simulink model "motorcontroller"  (R2015a)
settings: Solver=ode45  StartTime=0.0  StopTime=10.0  RelTol=1e-3
undefined symbols (not defined in the file): Hydride, magnitude, Metal, Nickel, Ts
libraries: powerlib x43, simulink_extras x8, driveline x4, electricdrivelib x3, simulink x2, powerlib_extras x2, DC6DriveInternalModels x1
(part 1 of 2)
settings Model: Creator=Elena  LastModifiedBy=Elena

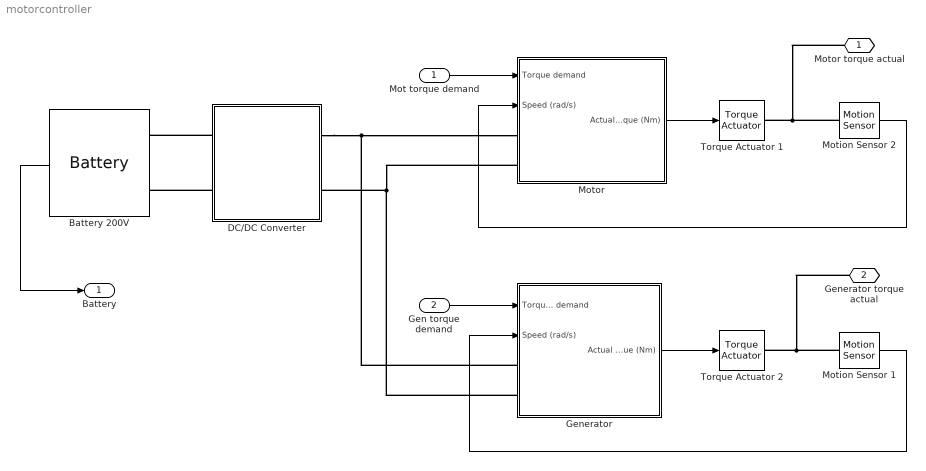
== system motorcontroller ==
  Mot torque demand : Inport
  Gen torque demand : Inport  Port=2
  Battery 200V : electricdrivelib/Extra Sources/Battery  BatType=Nickel-Metal-Hydride  ShowDetailedParameters=off  NomV=200  NomQ=6.5  SOC=final_SOC(end)  PresetModel=on  MaxQ=7  FullV=235.5932  Dis_rate=1.3  R=0.30769  Normal_OP=6.25  expZone="[216.9492           1.3]"  current=[50 100]  Units=Time  Batt_Tr=30
  DC/DC Converter : Subsystem
      mask init:
      | [X1,X1m,X2,X2m,X3,X4,Y1,Y1m,Y2,Y2m,Y3,Y4,color1,color2]=spsdrivelogo;
      mask Display:
      | patch([X1 X1m],[Y1 Y1m],color1);
      | patch(X3,Y3,color2);
      | plot([X1 X1m X2 X2m X3 X4],[Y1 Y1m Y2 Y2m Y3 Y4]);
  "Generator " : Subsystem
  Motion Sensor 1 : driveline/Sensors & Actuators/Motion Sensor  Angle=off  x0=0  Velocity=on  Acceleration=off
  Motion Sensor 2 : driveline/Sensors & Actuators/Motion Sensor  Angle=off  x0=0  Velocity=on  Acceleration=off
  Motor : Subsystem
  Torque Actuator 1 : driveline/Sensors & Actuators/Torque Actuator
  Torque Actuator 2 : driveline/Sensors & Actuators/Torque Actuator
  Motor torque actual : PMIOPort  Port=1  Side=Left
  Generator torque actual : PMIOPort  Port=2  Side=Right
  Battery : Outport
  wires:
  Battery 200V/1 -> Battery/1
  Mot torque demand/1 -> Motor/1(Torque demand)
  Gen torque demand/1 -> "Generator "/1(Torque demand)
  Motion Sensor 1/1 -> "Generator "/2(Speed (rad/s))
  Motor/1(Actual torque (Nm)) -> Torque Actuator 1/1
  "Generator "/1(Actual torque (Nm)) -> Torque Actuator 2/1
  Motion Sensor 2/1 -> Motor/2(Speed (rad/s))
  connections:
  DC/DC Converter/LConn1 -- Battery 200V/LConn1
  DC/DC Converter/LConn2 -- Battery 200V/LConn2
  DC/DC Converter/RConn1 -- "Generator "/LConn1 -- Motor/LConn1
  Motor/LConn2 -- "Generator "/LConn2 -- DC/DC Converter/RConn2
  Motor torque actual/RConn1 -- Motion Sensor 2/LConn1 -- Torque Actuator 1/RConn1
  Generator torque actual/RConn1 -- Torque Actuator 2/RConn1 -- Motion Sensor 1/LConn1

== system motorcontroller/DC//DC Converter ==
  Bus DC controller : Subsystem
  DC/DC converter : Subsystem
  Ubus Ref : Constant  Value=500
  +Vdc Bus : PMIOPort  Tag=PMCPort  Port=1  Side=Right
  -Vdc Bus : PMIOPort  Tag=PMCPort  Port=2  Side=Right
  + battery : PMIOPort  Tag=PMCPort  Port=3  Side=Left
  - battery : PMIOPort  Tag=PMCPort  Port=4  Side=Left
  wires:
  Ubus Ref/1 -> Bus DC controller/2(Uref)
  Bus DC controller/1(Duty cycle) -> DC/DC converter/1(Duty Cycle)
  DC/DC converter/1(UBus) -> Bus DC controller/1(Ubus)
  connections:
  +Vdc Bus/RConn1 -- DC/DC converter/LConn1
  -Vdc Bus/RConn1 -- DC/DC converter/LConn2
  + battery/RConn1 -- DC/DC converter/RConn1
  - battery/RConn1 -- DC/DC converter/RConn2

== system motorcontroller/Generator  ==
  Torque demand : Inport
  Speed (rad/s) : Inport  Port=2
  Bus Selector : BusSelector  OutputSignals=Rotor speed wm (rad/s),Rotor angle thetam (rad),Electromagnetic torque Te (N*m)
  Measures : electricdrivelib/AC drives/PM Synchronous Motor Drive/Measures
  Mux : Subsystem
  PMSM1 : powerlib/Machines/Permanent Magnet Synchronous Machine  NbPhases=3  FluxDistribution=Sinusoidal  RotorType=Salient-pole  MechanicalLoad=Speed w  PresetModel=No  ShowDetailedParameters=on  MeasurementBus=off  Resistance=0.05  Inductance=0  dqInductances=[0.000635 0.000635]  La=0.000835  MachineConstant=Flux linkage established by magnets (V.s)  Flux=0.192  VoltageCst=34.8249  TorqueCst=0.288  Flat=0  Mechanical=[0.011 0.001889/4 4/4]  PolePairs=1  InitialConditions=[0,0, 0,0,0]  InitialConditions5ph=[0 0 0 0 0 0]  TsPowergui=0  TsBlock=-1  RefAngle=90 degrees behind phase A axis (modified Park)
      settings: AttributesFormatString=\n
  Speed Controller : Subsystem  mask(Speed controller){SwK=Torque regulation, bs=1800, ramp=[-5000,5000], kp=(1/5)/4, ki=(50/5)/4/3, fc=(1000/10)/2, ctrl_sat=[-45,45], Tsc=Ts}
      mask prompts: SwK "Regulation type"; bs "Base speed (rpm)"; ramp "Speed reference ramp (rpm/s) [deceleration,acceleration]"; kp "Proportional gain"; ki "Integral gain"; fc "Speed measurement - low-pass filter cutoff frequency (Hz)"; ctrl_sat "Controller output torque saturation (N.m) [negative,positive]"; Tsc "Controller sampling time (s)"
      mask help: This block implements a PI speed regulator.
      mask init:
      | [X1,X1m,X2,X2m,X3,X4,Y1,Y1m,Y2,Y2m,Y3,Y4,color1,color2]=spsdrivelogo;
      mask TypeOptions SwK: Speed regulation | Torque regulation
      mask Display:
      | patch([X1 X1m],[Y1 Y1m],color1);
      | patch(X3,Y3,color2);
      | plot([X1 X1m X2 X2m X3 X4],[Y1 Y1m Y2 Y2m Y3 Y4]);
  Three-phase Inverter : Subsystem  mask(SPSdrives Converter){Arms=3, SnubberResistance=5000, SnubberCapacitance=inf, Device=IGBT / Diodes, Ron=1e-3, Lon=0, ForwardVoltages=[0.8,0.8], ForwardVoltage=0, GTOparameters=[0,0], IGBTparameters=[1e-6,2e-6], Measurements=All voltages and currents, SourceFrequency=60, dqInductances=[0.000635,0.000635], Flux=0.192, Resistance=0.05, p=4/4, converterType=Inverter}
      mask prompts: Arms "Number of bridge arms:"; SnubberResistance "Snubber resistance Rs (Ohms)"; SnubberCapacitance "Snubber capacitance Cs (F)"; Device "Power Electronic device"; Ron "Ron (Ohms)"; Lon "Lon (H)"; ForwardVoltages "Forward voltages  [ Device Vf(V) , Diode Vfd(V)]"; ForwardVoltage "Forward voltage Vf (V)"; GTOparameters "[  Tf (s) , Tt (s)  ]"; IGBTparameters "[  Tf (s) , Tt (s)  ]"; SourceFrequency "Source Frequency (Hz)"; dqInductances "PMSM-Inductances [ Ld(H) Lq(H) ]:"; Flux "PMSM-Flux induced by magnets (Wb):"; Resistance "PMSM-Stator resistance Rs (ohm):"; p "PMSM-Pairs of poles p:"; converterType "Converter type:"
      mask init:
      | Ld=dqInductances(1);
      | Lq=dqInductances(2);
      | Fcs=6*SourceFrequency/10;
      settings: OpenFcn=power_openblockproxy();
      mask Help: web(psbhelp);
      mask TypeOptions Arms: 1 | 2 | 3
      mask TypeOptions Device: Diodes | Thyristors | GTO / Diodes | MOSFET / Diodes | IGBT / Diodes | Ideal Switches
      mask TypeOptions Measurements: None | Device voltages | Device currents | UAB UBC UCA UDC voltages | All voltages and currents
      mask TypeOptions converterType: Rectifier | Inverter
      mask Display: plot(0,0,100,100,[39 39 23.8],[71 28 28],[44 56 49.6 56 52.8 56 61 61],[39.2 33.6 32.8 33.6 40.8 33.6 30 12.4],[44 44 44 61 61],[28 71 60 66.4 90],[75 67 83 75 67 83 75 75],[54 42 42 54 54 54 54 66],[61 75 75],[24 24 42],[75 75 61],[66,76,76])
  VECT : Subsystem  mask(VECT){nb_p=4/4, lambda=0.192, freq_max=20e3, Ts_vect=Ts, h=2}
      mask prompts: nb_p "Motor pairs of poles"; lambda "Flux induced by magnets (Wb)"; freq_max "Maximum switching frequency (Hz)"; Ts_vect "Sampling time (s)"; h "Current hysteresis bandwidth (A)"
      mask help: This block implements a vector controller.
      mask init:
      | [X1,X1m,X2,X2m,X3,X4,Y1,Y1m,Y2,Y2m,Y3,Y4,color1,color2]=spsdrivelogo;
      mask Display:
      | patch([X1 X1m],[Y1 Y1m],color1);
      | patch(X3,Y3,color2);
      | plot([X1 X1m X2 X2m X3 X4],[Y1 Y1m Y2 Y2m Y3 Y4]);
  + : PMIOPort  Port=1  Side=Left
  - : PMIOPort  Port=2  Side=Left
  Actual torque (Nm) : Outport
  wires:
  ? -> VECT/1(En), Speed Controller/3(En)
  Torque demand/1 -> Speed Controller/2(N*)
  Speed Controller/1(Torque*) -> VECT/2(Torque*)
  Bus Selector/1 -> Speed Controller/1(N)  "<Rotor speed wm (rad/s)>"
  PMSM1/1 -> Mux/2(m), Bus Selector/1
  Speed (rad/s)/1 -> PMSM1/1
  Bus Selector/3 -> Actual torque (Nm)/1  "<Electromagnetic torque Te (N*m)>"
  Measures/1 -> VECT/4(I_abc)
  Speed Controller/2(Ctrl) -> ?
  VECT/1(sig*) -> Mux/1(sig*)
  Mux/1(Ctrl) -> Three-phase Inverter/1(ctrl)
  Bus Selector/2 -> VECT/3(teta)  "<Rotor angle thetam (rad)>"
  connections:
  -/RConn1 -- Three-phase Inverter/RConn2
  +/RConn1 -- Three-phase Inverter/RConn1
  Measures/RConn1 -- PMSM1/LConn1
  Measures/RConn2 -- PMSM1/LConn2
  Measures/RConn3 -- PMSM1/LConn3
  Three-phase Inverter/LConn1 -- Measures/LConn1
  Measures/LConn2 -- Three-phase Inverter/LConn2
  Three-phase Inverter/LConn3 -- Measures/LConn3

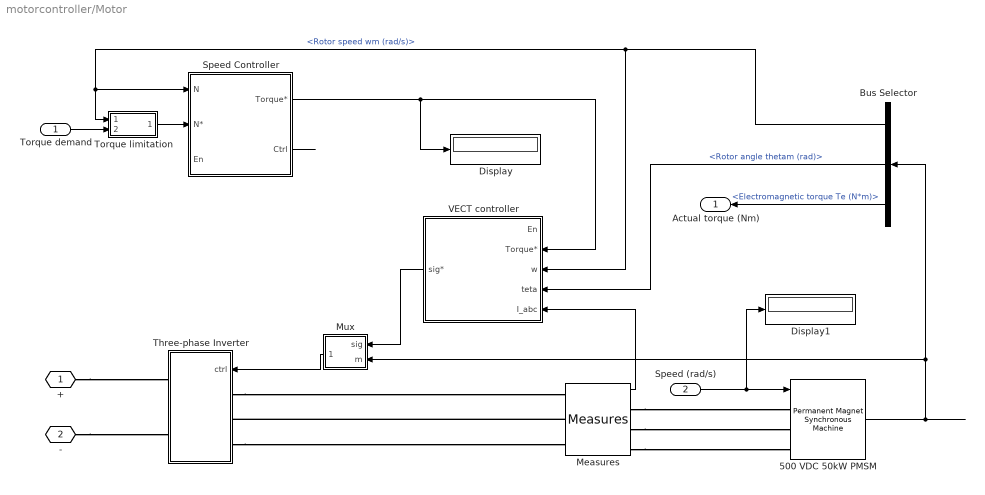
== system motorcontroller/Motor ==
  Torque demand : Inport
  Speed (rad/s) : Inport  Port=2
  500 VDC 50kW PMSM : powerlib/Machines/Permanent Magnet Synchronous Machine  NbPhases=3  FluxDistribution=Sinusoidal  RotorType=Salient-pole  MechanicalLoad=Speed w  PresetModel=No  ShowDetailedParameters=on  MeasurementBus=off  Resistance=0.0065  Inductance=0  dqInductances="[0.001597972349731   0.002057052250467]"  La=0.000835  MachineConstant=Flux linkage established by magnets (V.s)  Flux=0.175666143629361  VoltageCst=127.4493  TorqueCst=1.054  Flat=0  Mechanical=[0.089 0.005 4]  PolePairs=4  InitialConditions=[0,0,0,0]  InitialConditions5ph=[0 0 0 0 0 0]  TsPowergui=0  TsBlock=-1  RefAngle=90 degrees behind phase A axis (modified Park)
      settings: AttributesFormatString=\n
  Bus Selector : BusSelector  OutputSignals=Rotor speed wm (rad/s),Rotor angle thetam (rad),Electromagnetic torque Te (N*m)
  Display : Display
      settings: Decimation=100
  Display1 : Display
      settings: Decimation=100
  Measures : electricdrivelib/AC drives/PM Synchronous Motor Drive/Measures
  Mux : Subsystem
  Speed Controller : Subsystem  mask(Speed controller){SwK=Torque regulation, bs=3000, ramp=[-10000,10000], kp=1/5, ki=50/5, fc=1000/10, ctrl_sat=[-400,400], Tsc=120e-6}
      mask prompts: SwK "Regulation type"; bs "Base speed (rpm)"; ramp "Speed reference ramp (rpm/s) [deceleration,acceleration]"; kp "Proportional gain"; ki "Integral gain"; fc "Speed measurement - low-pass filter cutoff frequency (Hz)"; ctrl_sat "Controller output torque saturation (N.m) [negative,positive]"; Tsc "Controller sampling time (s)"
      mask help: This block implements a PI speed regulator.
      mask init:
      | [X1,X1m,X2,X2m,X3,X4,Y1,Y1m,Y2,Y2m,Y3,Y4,color1,color2]=spsdrivelogo;
      mask TypeOptions SwK: Speed regulation | Torque regulation
      mask Display:
      | patch([X1 X1m],[Y1 Y1m],color1);
      | patch(X3,Y3,color2);
      | plot([X1 X1m X2 X2m X3 X4],[Y1 Y1m Y2 Y2m Y3 Y4]);
  Three-phase Inverter : Subsystem  mask(SPSdrives Converter){Arms=3, SnubberResistance=5000, SnubberCapacitance=inf, Device=IGBT / Diodes, Ron=1e-3, Lon=0, ForwardVoltages=[0.8,0.8], ForwardVoltage=0, GTOparameters=[0,0], IGBTparameters=[1e-6,2e-6], Measurements=All voltages and currents, SourceFrequency=60, dqInductances=[0.001597972349731   0.002057052250467], Flux=0.175666143629361, Resistance=0.0065, p=4, converterType=Inverter}
      mask prompts: Arms "Number of bridge arms:"; SnubberResistance "Snubber resistance Rs (Ohms)"; SnubberCapacitance "Snubber capacitance Cs (F)"; Device "Power Electronic device"; Ron "Ron (Ohms)"; Lon "Lon (H)"; ForwardVoltages "Forward voltages  [ Device Vf(V) , Diode Vfd(V)]"; ForwardVoltage "Forward voltage Vf (V)"; GTOparameters "[  Tf (s) , Tt (s)  ]"; IGBTparameters "[  Tf (s) , Tt (s)  ]"; SourceFrequency "Source Frequency (Hz)"; dqInductances "PMSM-Inductances [ Ld(H) Lq(H) ]:"; Flux "PMSM-Flux induced by magnets (Wb):"; Resistance "PMSM-Stator resistance Rs (ohm):"; p "PMSM-Pairs of poles p:"; converterType "Converter type:"
      mask init:
      | Ld=dqInductances(1);
      | Lq=dqInductances(2);
      | Fcs=6*SourceFrequency/10;
      settings: OpenFcn=power_openblockproxy();
      mask Help: web(psbhelp);
      mask TypeOptions Arms: 1 | 2 | 3
      mask TypeOptions Device: Diodes | Thyristors | GTO / Diodes | MOSFET / Diodes | IGBT / Diodes | Ideal Switches
      mask TypeOptions Measurements: None | Device voltages | Device currents | UAB UBC UCA UDC voltages | All voltages and currents
      mask TypeOptions converterType: Rectifier | Inverter
      mask Display: plot(0,0,100,100,[39 39 23.8],[71 28 28],[44 56 49.6 56 52.8 56 61 61],[39.2 33.6 32.8 33.6 40.8 33.6 30 12.4],[44 44 44 61 61],[28 71 60 66.4 90],[75 67 83 75 67 83 75 75],[54 42 42 54 54 54 54 66],[61 75 75],[24 24 42],[75 75 61],[66,76,76])
  Torque limitation : Subsystem
      mask Display: plot([0;1800;2000;2500;3000;3500], [1;1;0.90*1;0.72*1;0.6*1;0.51*1])
  VECT controller : Subsystem  mask(VECT){nb_p=4, dqInductances=[0.001597972349731   0.002057052250467], lambda=0.175666143629361, Ts_vect=60e-6}
      mask prompts: nb_p "Motor pairs of poles"; dqInductances "Inductances [ Ld(H) Lq(H) ]:"; lambda "Flux induced by magnets (Wb)"; Ts_vect "Sampling time (s)"
      mask help: This block implements a vector controller.
      mask init:
      | [X1,X1m,X2,X2m,X3,X4,Y1,Y1m,Y2,Y2m,Y3,Y4,color1,color2]=spsdrivelogo;
      | ib = lambda/(dqInductances(2)-dqInductances(1));
      | Teb = 3/2*nb_p*lambda*ib;
      | Ld = dqInductances(1);
      | Lq = dqInductances(2);
      | lam = lambda;
      | p=nb_p;
      | ib = lam/(Lq-Ld);
      | iqn = 0:0.01:3;
      | ten = iqn/2.*(sqrt(4*iqn.*iqn+1)+1);
      mask Display:
      | patch([X1 X1m],[Y1 Y1m],color1);
      | patch(X3,Y3,color2);
      | plot([X1 X1m X2 X2m X3 X4],[Y1 Y1m Y2 Y2m Y3 Y4]);
  + : PMIOPort  Port=1  Side=Left
  - : PMIOPort  Port=2  Side=Left
  Actual torque (Nm) : Outport
  wires:
  Mux/1(Ctrl) -> Three-phase Inverter/1(ctrl)
  VECT controller/1(sig*) -> Mux/1(sig)
  Speed Controller/2(Ctrl) -> ?
  Speed (rad/s)/1 -> Display1/1, 500 VDC 50kW PMSM/1
  500 VDC 50kW PMSM/1 -> Bus Selector/1, Mux/2(m)
  Bus Selector/3 -> Actual torque (Nm)/1  "<Electromagnetic torque Te (N*m)>"
  Bus Selector/1 -> VECT controller/3(w), Speed Controller/1(N), Torque limitation/1(N rad/s)  "<Rotor speed wm (rad/s)>"
  ? -> VECT controller/1(En), Speed Controller/3(En)
  Speed Controller/1(Torque*) -> Display/1, VECT controller/2(Torque*)
  Measures/1 -> VECT controller/5(I_abc)
  Bus Selector/2 -> VECT controller/4(teta)  "<Rotor angle thetam (rad)>"
  Torque limitation/1(torque) -> Speed Controller/2(N*)
  Torque demand/1 -> Torque limitation/2(Torque)
  connections:
  Three-phase Inverter/LConn3 -- Measures/LConn3
  Measures/LConn2 -- Three-phase Inverter/LConn2
  Three-phase Inverter/LConn1 -- Measures/LConn1
  Measures/RConn3 -- 500 VDC 50kW PMSM/LConn3
  Measures/RConn2 -- 500 VDC 50kW PMSM/LConn2
  Measures/RConn1 -- 500 VDC 50kW PMSM/LConn1
  +/RConn1 -- Three-phase Inverter/RConn1
  -/RConn1 -- Three-phase Inverter/RConn2

== system motorcontroller/DC//DC Converter/Bus DC controller ==
  Ubus : Inport
  Uref : Inport  Port=2
  Current controller DISCRETE1 : Subsystem  mask(PI controller){Kp=0.001, Ki=1, Ts=Ts}
      mask prompts: Kp "Proportional gain (Kp)"; Ki "Integral gain (Ki)"; Ts "Sample time (s) :"
      mask help: Proportional-Integral Speed Controller
      mask Display: plot(0,0,100,100,[35,35,65],[70,30,30],[35,65],[45,60])
  Display : Display
      settings: Decimation=100
  Duty Cycles : Subsystem
  Mux : Mux  Inputs=2
  Unit Delay2 : UnitDelay  InitialCondition=.5  SampleTime=Ts
  Zero-Order Hold1 : ZeroOrderHold  SampleTime=Ts
  Duty cycle : Outport  InitialOutput=0
  tag scope: V_DCDC=global
  wires:
  Ubus/1 -> Mux/2, Zero-Order Hold1/1
  Mux/1 -> [V_DCDC]
  Uref/1 -> Current controller DISCRETE1/2(Uref), Mux/1
  Current controller DISCRETE1/1(Ec) -> Duty Cycles/1(Ec)
  Zero-Order Hold1/1 -> Display/1, Current controller DISCRETE1/1(UBus)
  Duty Cycles/1(dc) -> Unit Delay2/1
  Unit Delay2/1 -> Duty cycle/1

== system motorcontroller/DC//DC Converter/DC//DC converter ==
  Duty Cycle : Inport
  CBus : powerlib/Elements/Series RLC Branch  LConnTagsString=__new0  RConnTagsString=__new0  BranchType=RC  Resistance=0.2  Inductance=1e-3  SetiL0=off  InitialCurrent=0  Capacitance=1130e-6  Setx0=on  InitialVoltage=500  Measurements=None
  CBus1 : powerlib/Elements/Series RLC Branch  LConnTagsString=__new0  RConnTagsString=__new0  BranchType=C  Resistance=0.2  Inductance=1e-3  SetiL0=off  InitialCurrent=0  Capacitance=282e-6  Setx0=on  InitialVoltage=150  Measurements=None
  Chopper : DC6DriveInternalModels/Chopper (average model)  SnubberResistance=10e3  SnubberCapacitance=inf  Ron=1e-3  ForwardVoltages=[1.3,1.3]  IGBTParameters=[0,0]  converterType=Inverter
  L : powerlib/Elements/Series RLC Branch  LConnTagsString=__new0  RConnTagsString=__new0  BranchType=L  Resistance=0.3  Inductance=373e-6  SetiL0=off  InitialCurrent=100  Capacitance=100e-6  Setx0=off  InitialVoltage=0  Measurements=None
  Neutral2 : powerlib/Elements/Neutral  LConnTagsString=a  NodeNumber=10
  V1 : powerlib/Measurements/Voltage Measurement  PhasorSimulation=off  OutputType=Complex  PSBequivalent=0
  + : PMIOPort  Tag=PMCPort  Port=1  Side=Left
  - : PMIOPort  Tag=PMCPort  Port=2  Side=Left
  + bat. : PMIOPort  Tag=PMCPort  Port=3  Side=Right
  - bat. : PMIOPort  Tag=PMCPort  Port=4  Side=Right
  UBus : Outport
  wires:
  Duty Cycle/1 -> Chopper/1
  V1/1 -> UBus/1
  connections:
  Chopper/RConn1 -- L/RConn1
  L/LConn1 -- + bat./RConn1 -- CBus1/LConn1
  CBus1/RConn1 -- - bat./RConn1 -- Chopper/LConn2 -- -/RConn1 -- CBus/RConn1 -- V1/LConn2 -- Neutral2/LConn1
  +/RConn1 -- CBus/LConn1 -- Chopper/LConn1 -- V1/LConn1

== system motorcontroller/Generator /Mux ==
  sig* : Inport
  m : Inport  Port=2
  Bus Creator : BusCreator  Inputs=2
  Ctrl : Outport
  wires:
  m/1 -> Bus Creator/2  "m"
  sig*/1 -> Bus Creator/1  "Signals*"
  Bus Creator/1 -> Ctrl/1

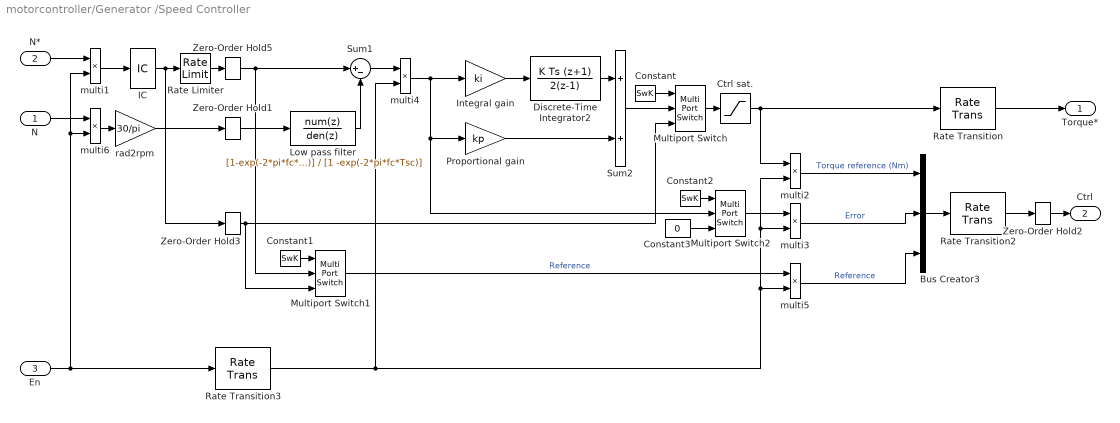
== system motorcontroller/Generator /Speed Controller ==
  N : Inport
  N* : Inport  Port=2
  En : Inport  Port=3
  Bus Creator3 : BusCreator  Inputs=3
  Constant : Constant  Value=SwK
  Constant1 : Constant  Value=SwK
  Constant2 : Constant  Value=SwK
  Constant3 : Constant  Value=0
  Ctrl sat. : Saturate  UpperLimit=ctrl_sat(2)  LowerLimit=ctrl_sat(1)
  Discrete-Time Integrator2 : DiscreteIntegrator  IntegratorMethod=Integration: Trapezoidal  SampleTime=Tsc  LimitOutput=on  UpperSaturationLimit=ctrl_sat(2)  LowerSaturationLimit=ctrl_sat(1)
  IC : InitialCondition  Value=0
  Integral gain : Gain  Gain=ki  SaturateOnIntegerOverflow=on  OutDataTypeStr=Inherit: Same as input  ParamDataTypeStr=Inherit: Same as input
  Low pass filter : DiscreteTransferFcn  Numerator=[1-exp(-2*pi*fc*Tsc)]  Denominator=[1 -exp(-2*pi*fc*Tsc)]  SampleTime=Tsc
  Multiport Switch : MultiPortSwitch  Inputs=2  SaturateOnIntegerOverflow=on
  Multiport Switch1 : MultiPortSwitch  Inputs=2  SaturateOnIntegerOverflow=on
  Multiport Switch2 : MultiPortSwitch  Inputs=2  SaturateOnIntegerOverflow=on
  Proportional gain : Gain  Gain=kp  SaturateOnIntegerOverflow=on  OutDataTypeStr=Inherit: Same as input  ParamDataTypeStr=Inherit: Same as input
  Rate Limiter : RateLimiter  RisingSlewLimit=ramp(2)  FallingSlewLimit=ramp(1)  LinearizeAsGain=off
  Rate Transition : RateTransition
  Rate Transition2 : RateTransition
  Rate Transition3 : RateTransition
  Sum1 : Sum  Inputs=|+-  SaturateOnIntegerOverflow=on  InputSameDT=on  OutDataTypeStr=Inherit: Same as first input
  Sum2 : Sum  SaturateOnIntegerOverflow=on  InputSameDT=on  OutDataTypeStr=Inherit: Same as first input
  Zero-Order Hold1 : ZeroOrderHold  SampleTime=Tsc
  Zero-Order Hold2 : ZeroOrderHold  SampleTime=Ts
  Zero-Order Hold3 : ZeroOrderHold  SampleTime=Tsc
  Zero-Order Hold5 : ZeroOrderHold  SampleTime=Tsc
  multi{1..6} (6 alike) : Product
  rad2rpm : Gain  Gain=30/pi  SaturateOnIntegerOverflow=on  OutDataTypeStr=Inherit: Same as input  ParamDataTypeStr=Inherit: Same as input
  Torque* : Outport
  Ctrl : Outport  Port=2
  wires:
  N/1 -> multi6/1
  multi6/1 -> rad2rpm/1
  N*/1 -> multi1/1
  multi1/1 -> IC/1
  Rate Transition3/1 -> multi5/2, multi2/2, multi3/2, multi4/2
  multi4/1 -> Multiport Switch2/2, Proportional gain/1, Integral gain/1
  Low pass filter/1 -> Sum1/2
  multi2/1 -> Bus Creator3/1  "Torque reference (Nm)"
  Multiport Switch1/1 -> multi5/1  "Reference"
  multi5/1 -> Bus Creator3/3  "Reference"
  multi3/1 -> Bus Creator3/2  "Error"
  Multiport Switch2/1 -> multi3/1
  Zero-Order Hold2/1 -> Ctrl/1
  Rate Transition/1 -> Torque*/1
  En/1 -> multi6/2, multi1/2, Rate Transition3/1
  rad2rpm/1 -> Zero-Order Hold1/1
  Constant3/1 -> Multiport Switch2/3
  Constant2/1 -> Multiport Switch2/1
  Zero-Order Hold3/1 -> Multiport Switch1/3, Multiport Switch/3
  Constant1/1 -> Multiport Switch1/1
  Sum2/1 -> Multiport Switch/2
  Constant/1 -> Multiport Switch/1
  Multiport Switch/1 -> Ctrl sat./1
  Zero-Order Hold5/1 -> Multiport Switch1/2, Sum1/1
  Rate Limiter/1 -> Zero-Order Hold5/1
  Bus Creator3/1 -> Rate Transition2/1
  Rate Transition2/1 -> Zero-Order Hold2/1
  Zero-Order Hold1/1 -> Low pass filter/1
  IC/1 -> Zero-Order Hold3/1, Rate Limiter/1
  Proportional gain/1 -> Sum2/2
  Discrete-Time Integrator2/1 -> Sum2/1
  Sum1/1 -> multi4/1
  Integral gain/1 -> Discrete-Time Integrator2/1
  Ctrl sat./1 -> multi2/1, Rate Transition/1

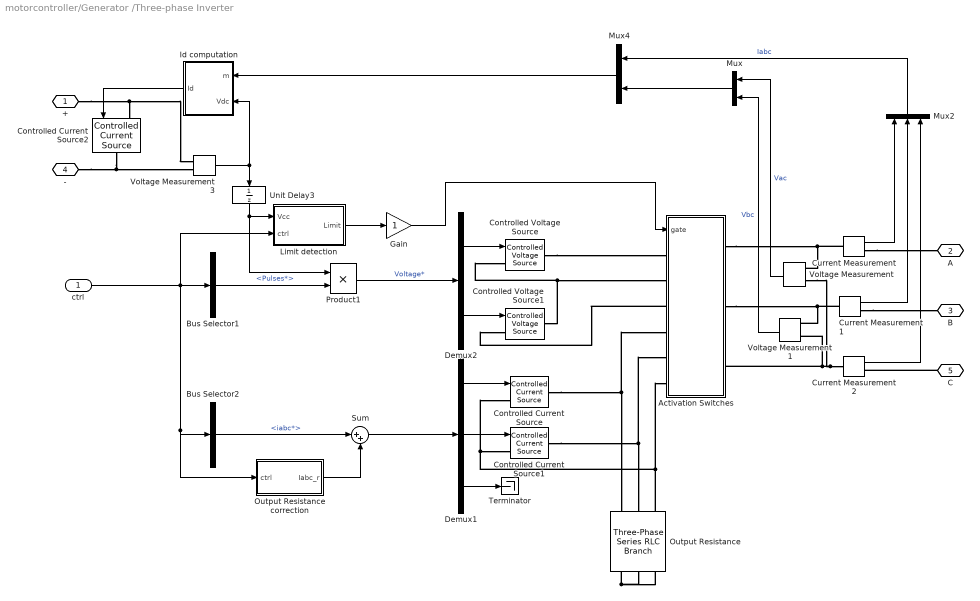
== system motorcontroller/Generator /Three-phase Inverter ==
  ctrl : Inport
  Activation Switches : Subsystem
  Bus Selector1 : BusSelector  OutputSignals=Signals*.Pulses*
  Bus Selector2 : BusSelector  OutputSignals=Signals*.iabc*
  Controlled Current Source : powerlib/Electrical Sources/Controlled Current Source  Initialize=on  Source_Type=AC  Amplitude=0  Phase=0  Frequency=0  Measurements=None
  Controlled Current Source1 : powerlib/Electrical Sources/Controlled Current Source  Initialize=on  Source_Type=AC  Amplitude=0  Phase=0  Frequency=0  Measurements=None
  Controlled Current Source2 : powerlib/Electrical Sources/Controlled Current Source  Initialize=on  Source_Type=AC  Amplitude=0  Phase=0  Frequency=0  Measurements=None
  Controlled Voltage Source : powerlib/Electrical Sources/Controlled Voltage Source  Initialize=on  Source_Type=AC  Amplitude=0  Phase=0  Frequency=0  Measurements=None
  Controlled Voltage Source1 : powerlib/Electrical Sources/Controlled Voltage Source  Initialize=on  Source_Type=AC  Amplitude=0  Phase=0  Frequency=0  Measurements=None
  Current Measurement : powerlib/Measurements/Current Measurement  PhasorSimulation=off  OutputType=Complex  PSBequivalent=0
  Current Measurement1 : powerlib/Measurements/Current Measurement  PhasorSimulation=off  OutputType=Complex  PSBequivalent=0
  Current Measurement2 : powerlib/Measurements/Current Measurement  PhasorSimulation=off  OutputType=Complex  PSBequivalent=0
  Demux1 : Demux  Outputs=3
  Demux2 : Demux  Outputs=2
  Gain : Gain
  Id computation : Subsystem
  Limit detection : Subsystem
  Mux : Mux  Inputs=2
  Mux2 : Mux  Inputs=3
  Mux4 : Mux  Inputs=2
  Output Resistance : powerlib/Elements/Three-Phase Series RLC Branch  LConnTagsString=A|B|C  RConnTagsString=A|B|C  BranchType=R  Resistance=100*Resistance  Inductance=1e-3  Capacitance=1e-6  Measurements=Branch voltages and currents
  Output Resistance correction : Subsystem
  Product1 : Product  RndMeth=Zero
  Sum : Sum  Inputs=|++
  Terminator : Terminator
  Unit Delay3 : UnitDelay  SampleTime=Ts
  Voltage Measurement : powerlib/Measurements/Voltage Measurement  PhasorSimulation=off  OutputType=Complex  PSBequivalent=0
  Voltage Measurement1 : powerlib/Measurements/Voltage Measurement  PhasorSimulation=off  OutputType=Complex  PSBequivalent=0
  Voltage Measurement3 : powerlib/Measurements/Voltage Measurement  PhasorSimulation=off  OutputType=Complex  PSBequivalent=0
  + : PMIOPort  Port=1  Side=Right
  A : PMIOPort  Port=2  Side=Left
  B : PMIOPort  Port=3  Side=Left
  - : PMIOPort  Port=4  Side=Right
  C : PMIOPort  Port=5  Side=Left
  wires:
  Gain/1 -> Activation Switches/1(gate)
  Output Resistance correction/1("Iabc_r ") -> Sum/2
  Product1/1 -> Demux2/1  "Voltage*"
  ctrl/1 -> Output Resistance correction/1(ctrl), Bus Selector2/1, Limit detection/2(ctrl), Bus Selector1/1
  Unit Delay3/1 -> Limit detection/1(Vcc), Product1/1
  Sum/1 -> Demux1/1
  Limit detection/1(Limit) -> Gain/1
  Bus Selector2/1 -> Sum/1  "<iabc*>"
  Demux2/1 -> Controlled Voltage Source/1
  Demux2/2 -> Controlled Voltage Source1/1
  Demux1/3 -> Terminator/1
  Demux1/2 -> Controlled Current Source1/1
  Demux1/1 -> Controlled Current Source/1
  Bus Selector1/1 -> Product1/2  "<Pulses*>"
  Voltage Measurement3/1 -> Id computation/2(Vdc), Unit Delay3/1
  Id computation/1(Id) -> Controlled Current Source2/1
  Mux2/1 -> Mux4/1  "Iabc"
  Mux4/1 -> Id computation/1(m)
  Current Measurement2/1 -> Mux2/3
  Mux/1 -> Mux4/2
  Voltage Measurement1/1 -> Mux/2  "Vbc"
  Voltage Measurement/1 -> Mux/1  "Vac"
  Current Measurement1/1 -> Mux2/2
  Current Measurement/1 -> Mux2/1
  connections:
  Activation Switches/LConn3 -- Controlled Voltage Source1/LConn1
  Controlled Voltage Source/RConn1 -- Activation Switches/LConn1
  C/RConn1 -- Current Measurement2/RConn1
  Current Measurement1/RConn1 -- B/RConn1
  Current Measurement/RConn1 -- A/RConn1
  Current Measurement1/LConn1 -- Activation Switches/RConn2 -- Voltage Measurement1/LConn1
  Controlled Voltage Source1/RConn1 -- Activation Switches/LConn2 -- Controlled Voltage Source/LConn1
  Current Measurement2/LConn1 -- Voltage Measurement1/LConn2 -- Activation Switches/RConn3 -- Voltage Measurement/LConn2
  Controlled Current Source1/RConn1 -- Activation Switches/LConn5 -- Output Resistance/LConn2
  Controlled Current Source/RConn1 -- Activation Switches/LConn4 -- Output Resistance/LConn1
  Current Measurement/LConn1 -- Activation Switches/RConn1 -- Voltage Measurement/LConn1
  Output Resistance/RConn1 -- Output Resistance/RConn2 -- Output Resistance/RConn3
  Output Resistance/LConn3 -- Controlled Current Source1/LConn1 -- Controlled Current Source/LConn1 -- Activation Switches/LConn6
  -/RConn1 -- Controlled Current Source2/RConn1 -- Voltage Measurement3/LConn2
  +/RConn1 -- Controlled Current Source2/LConn1 -- Voltage Measurement3/LConn1

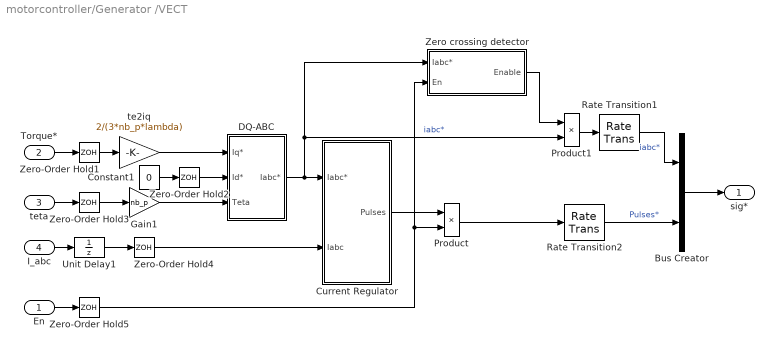
== system motorcontroller/Generator /VECT ==
  En : Inport
  Torque* : Inport  Port=2
  teta : Inport  Port=3
  I_abc : Inport  Port=4
  Bus Creator : BusCreator  Inputs=2
  Constant1 : Constant  Value=0
  Current Regulator : Subsystem
  DQ-ABC : Subsystem
  Gain1 : Gain  Gain=nb_p  SaturateOnIntegerOverflow=on  OutDataTypeStr=Inherit: Same as input  ParamDataTypeStr=Inherit: Same as input
  Product : Product  RndMeth=Zero
  Product1 : Product  RndMeth=Zero
  Rate Transition1 : RateTransition
  Rate Transition2 : RateTransition
  Unit Delay1 : UnitDelay  SampleTime=Ts
  Zero crossing detector : Subsystem
  Zero-Order Hold{1..5} (5 alike) : ZeroOrderHold  SampleTime=Ts_vect
  te2iq : Gain  Gain=2/(3*nb_p*lambda)  SaturateOnIntegerOverflow=on  OutDataTypeStr=Inherit: Same as input  ParamDataTypeStr=Inherit: Same as input
  sig* : Outport
  wires:
  Zero-Order Hold5/1 -> Zero crossing detector/2(En), Product/2
  Zero crossing detector/1(Enable) -> Product1/1
  En/1 -> Zero-Order Hold5/1
  Product1/1 -> Rate Transition1/1
  Product/1 -> Rate Transition2/1
  Current Regulator/1(Pulses) -> Product/1
  Zero-Order Hold4/1 -> Current Regulator/2(Iabc)
  Rate Transition1/1 -> Bus Creator/1  "iabc*"
  Rate Transition2/1 -> Bus Creator/2  "Pulses*"
  Bus Creator/1 -> sig*/1
  te2iq/1 -> DQ-ABC/1("Iq* ")
  Zero-Order Hold2/1 -> DQ-ABC/2("Id* ")
  Zero-Order Hold1/1 -> te2iq/1
  teta/1 -> Zero-Order Hold3/1
  Zero-Order Hold3/1 -> Gain1/1
  Torque*/1 -> Zero-Order Hold1/1
  Constant1/1 -> Zero-Order Hold2/1
  Gain1/1 -> DQ-ABC/3(Teta)
  Unit Delay1/1 -> Zero-Order Hold4/1
  DQ-ABC/1(Iabc*) -> Zero crossing detector/1(Iabc*), Product1/2, Current Regulator/1(Iabc*)  "iabc*"
  I_abc/1 -> Unit Delay1/1

== system motorcontroller/Motor/Mux ==
  sig : Inport
  m : Inport  Port=2
  Bus Creator : BusCreator  Inputs=2
  Ctrl : Outport
  wires:
  Bus Creator/1 -> Ctrl/1
  sig/1 -> Bus Creator/1  "sig"
  m/1 -> Bus Creator/2  "m"

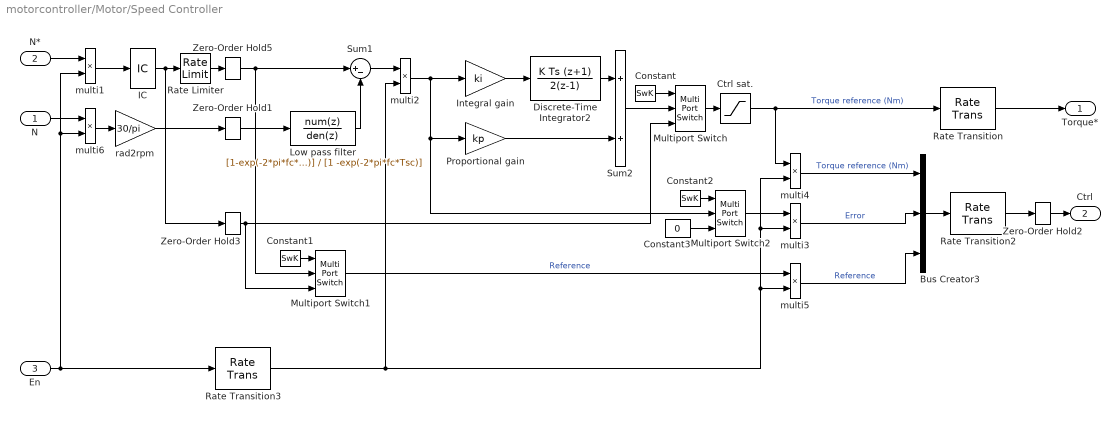
== system motorcontroller/Motor/Speed Controller ==
  N : Inport
  N* : Inport  Port=2
  En : Inport  Port=3
  Bus Creator3 : BusCreator  Inputs=3
  Constant : Constant  Value=SwK
  Constant1 : Constant  Value=SwK
  Constant2 : Constant  Value=SwK
  Constant3 : Constant  Value=0
  Ctrl sat. : Saturate  UpperLimit=ctrl_sat(2)  LowerLimit=ctrl_sat(1)
  Discrete-Time Integrator2 : DiscreteIntegrator  IntegratorMethod=Integration: Trapezoidal  SampleTime=Tsc  LimitOutput=on  UpperSaturationLimit=ctrl_sat(2)  LowerSaturationLimit=ctrl_sat(1)
  IC : InitialCondition  Value=0
  Integral gain : Gain  Gain=ki  SaturateOnIntegerOverflow=on  OutDataTypeStr=Inherit: Same as input  ParamDataTypeStr=Inherit: Same as input
  Low pass filter : DiscreteTransferFcn  Numerator=[1-exp(-2*pi*fc*Tsc)]  Denominator=[1 -exp(-2*pi*fc*Tsc)]  SampleTime=Tsc
  Multiport Switch : MultiPortSwitch  Inputs=2  SaturateOnIntegerOverflow=on
  Multiport Switch1 : MultiPortSwitch  Inputs=2  SaturateOnIntegerOverflow=on
  Multiport Switch2 : MultiPortSwitch  Inputs=2  SaturateOnIntegerOverflow=on
  Proportional gain : Gain  Gain=kp  SaturateOnIntegerOverflow=on  OutDataTypeStr=Inherit: Same as input  ParamDataTypeStr=Inherit: Same as input
  Rate Limiter : RateLimiter  RisingSlewLimit=ramp(2)  FallingSlewLimit=ramp(1)  LinearizeAsGain=off
  Rate Transition : RateTransition
  Rate Transition2 : RateTransition
  Rate Transition3 : RateTransition
  Sum1 : Sum  Inputs=|+-  SaturateOnIntegerOverflow=on  InputSameDT=on  OutDataTypeStr=Inherit: Same as first input
  Sum2 : Sum  SaturateOnIntegerOverflow=on  InputSameDT=on  OutDataTypeStr=Inherit: Same as first input
  Zero-Order Hold1 : ZeroOrderHold  SampleTime=Tsc
  Zero-Order Hold2 : ZeroOrderHold  SampleTime=Ts
  Zero-Order Hold3 : ZeroOrderHold  SampleTime=Tsc
  Zero-Order Hold5 : ZeroOrderHold  SampleTime=Tsc
  multi{1..6} (6 alike) : Product
  rad2rpm : Gain  Gain=30/pi  SaturateOnIntegerOverflow=on  OutDataTypeStr=Inherit: Same as input  ParamDataTypeStr=Inherit: Same as input
  Torque* : Outport
  Ctrl : Outport  Port=2
  wires:
  Ctrl sat./1 -> multi4/1, Rate Transition/1  "Torque reference (Nm)"
  Integral gain/1 -> Discrete-Time Integrator2/1
  Sum1/1 -> multi2/1
  Discrete-Time Integrator2/1 -> Sum2/1
  Proportional gain/1 -> Sum2/2
  IC/1 -> Rate Limiter/1, Zero-Order Hold3/1
  Zero-Order Hold1/1 -> Low pass filter/1
  Rate Transition2/1 -> Zero-Order Hold2/1
  Bus Creator3/1 -> Rate Transition2/1
  Low pass filter/1 -> Sum1/2
  Rate Limiter/1 -> Zero-Order Hold5/1
  Zero-Order Hold5/1 -> Sum1/1, Multiport Switch1/2
  Multiport Switch/1 -> Ctrl sat./1
  Constant/1 -> Multiport Switch/1
  Sum2/1 -> Multiport Switch/2
  Constant1/1 -> Multiport Switch1/1
  Zero-Order Hold3/1 -> Multiport Switch/3, Multiport Switch1/3
  Constant2/1 -> Multiport Switch2/1
  Constant3/1 -> Multiport Switch2/3
  rad2rpm/1 -> Zero-Order Hold1/1
  En/1 -> Rate Transition3/1, multi1/2, multi6/2
  Rate Transition/1 -> Torque*/1
  Zero-Order Hold2/1 -> Ctrl/1
  Multiport Switch2/1 -> multi3/1
  multi3/1 -> Bus Creator3/2  "Error"
  multi5/1 -> Bus Creator3/3  "Reference"
  Multiport Switch1/1 -> multi5/1  "Reference"
  multi4/1 -> Bus Creator3/1  "Torque reference (Nm)"
  multi2/1 -> Integral gain/1, Proportional gain/1, Multiport Switch2/2
  Rate Transition3/1 -> multi2/2, multi4/2, multi3/2, multi5/2
  multi6/1 -> rad2rpm/1
  multi1/1 -> IC/1
  N*/1 -> multi1/1
  N/1 -> multi6/1

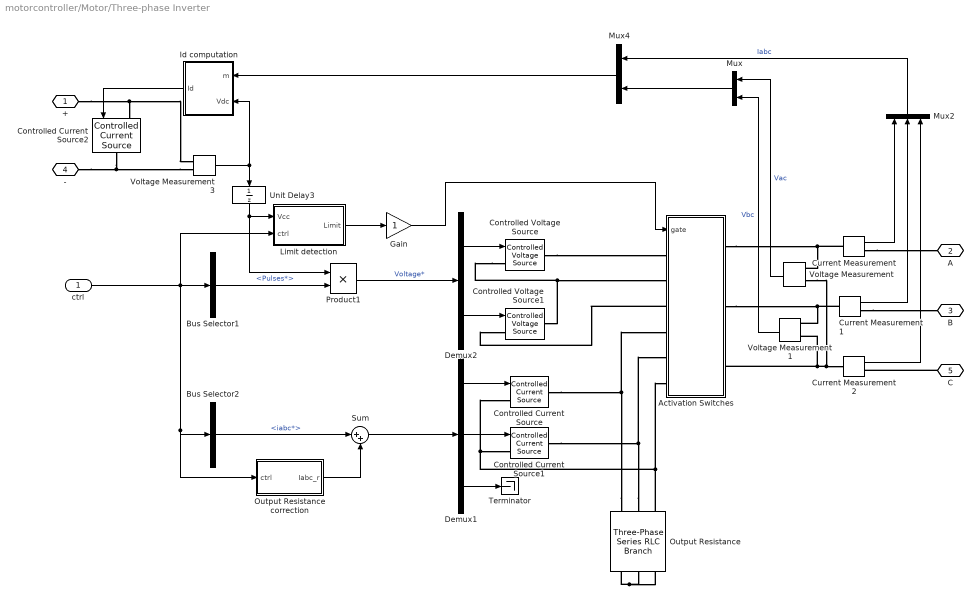
== system motorcontroller/Motor/Three-phase Inverter ==
  ctrl : Inport
  Activation Switches : Subsystem
  Bus Selector1 : BusSelector  OutputSignals=sig.Pulses*
  Bus Selector2 : BusSelector  OutputSignals=sig.iabc*
  Controlled Current Source : powerlib/Electrical Sources/Controlled Current Source  Initialize=on  Source_Type=AC  Amplitude=0  Phase=0  Frequency=0  Measurements=None
  Controlled Current Source1 : powerlib/Electrical Sources/Controlled Current Source  Initialize=on  Source_Type=AC  Amplitude=0  Phase=0  Frequency=0  Measurements=None
  Controlled Current Source2 : powerlib/Electrical Sources/Controlled Current Source  Initialize=on  Source_Type=AC  Amplitude=0  Phase=0  Frequency=0  Measurements=None
  Controlled Voltage Source : powerlib/Electrical Sources/Controlled Voltage Source  Initialize=on  Source_Type=AC  Amplitude=0  Phase=0  Frequency=0  Measurements=None
  Controlled Voltage Source1 : powerlib/Electrical Sources/Controlled Voltage Source  Initialize=on  Source_Type=AC  Amplitude=0  Phase=0  Frequency=0  Measurements=None
  Current Measurement : powerlib/Measurements/Current Measurement  PhasorSimulation=off  OutputType=Complex  PSBequivalent=0
  Current Measurement1 : powerlib/Measurements/Current Measurement  PhasorSimulation=off  OutputType=Complex  PSBequivalent=0
  Current Measurement2 : powerlib/Measurements/Current Measurement  PhasorSimulation=off  OutputType=Complex  PSBequivalent=0
  Demux1 : Demux  Outputs=3
  Demux2 : Demux  Outputs=2
  Gain : Gain
  Id computation : Subsystem
  Limit detection : Subsystem
  Mux : Mux  Inputs=2
  Mux2 : Mux  Inputs=3
  Mux4 : Mux  Inputs=2
  Output Resistance : powerlib/Elements/Three-Phase Series RLC Branch  LConnTagsString=A|B|C  RConnTagsString=A|B|C  BranchType=R  Resistance=100*Resistance  Inductance=1e-3  Capacitance=1e-6  Measurements=Branch voltages and currents
  Output Resistance correction : Subsystem
  Product1 : Product  RndMeth=Zero
  Sum : Sum  Inputs=|++
  Terminator : Terminator
  Unit Delay3 : UnitDelay  SampleTime=Ts
  Voltage Measurement : powerlib/Measurements/Voltage Measurement  PhasorSimulation=off  OutputType=Complex  PSBequivalent=0
  Voltage Measurement1 : powerlib/Measurements/Voltage Measurement  PhasorSimulation=off  OutputType=Complex  PSBequivalent=0
  Voltage Measurement3 : powerlib/Measurements/Voltage Measurement  PhasorSimulation=off  OutputType=Complex  PSBequivalent=0
  + : PMIOPort  Port=1  Side=Right
  A : PMIOPort  Port=2  Side=Left
  B : PMIOPort  Port=3  Side=Left
  - : PMIOPort  Port=4  Side=Right
  C : PMIOPort  Port=5  Side=Left
  wires:
  Current Measurement/1 -> Mux2/1
  Current Measurement1/1 -> Mux2/2
  Voltage Measurement/1 -> Mux/1  "Vac"
  Voltage Measurement1/1 -> Mux/2  "Vbc"
  Mux/1 -> Mux4/2
  Current Measurement2/1 -> Mux2/3
  Mux4/1 -> Id computation/1(m)
  Mux2/1 -> Mux4/1  "Iabc"
  Voltage Measurement3/1 -> Unit Delay3/1, Id computation/2(Vdc)
  Bus Selector1/1 -> Product1/2  "<Pulses*>"
  Demux1/1 -> Controlled Current Source/1
  Demux1/2 -> Controlled Current Source1/1
  Demux1/3 -> Terminator/1
  Demux2/2 -> Controlled Voltage Source1/1
  Demux2/1 -> Controlled Voltage Source/1
  Bus Selector2/1 -> Sum/1  "<iabc*>"
  Limit detection/1(Limit) -> Gain/1
  Sum/1 -> Demux1/1
  Unit Delay3/1 -> Product1/1, Limit detection/1(Vcc)
  ctrl/1 -> Bus Selector1/1, Limit detection/2(ctrl), Bus Selector2/1, Output Resistance correction/1(ctrl)
  Product1/1 -> Demux2/1  "Voltage*"
  Gain/1 -> Activation Switches/1(gate)
  Id computation/1(Id) -> Controlled Current Source2/1
  Output Resistance correction/1("Iabc_r ") -> Sum/2
  connections:
  Voltage Measurement3/LConn1 -- Controlled Current Source2/LConn1 -- +/RConn1
  Voltage Measurement3/LConn2 -- Controlled Current Source2/RConn1 -- -/RConn1
  Activation Switches/LConn6 -- Controlled Current Source/LConn1 -- Controlled Current Source1/LConn1 -- Output Resistance/LConn3
  Output Resistance/RConn3 -- Output Resistance/RConn2 -- Output Resistance/RConn1
  Voltage Measurement/LConn1 -- Activation Switches/RConn1 -- Current Measurement/LConn1
  Output Resistance/LConn1 -- Activation Switches/LConn4 -- Controlled Current Source/RConn1
  Output Resistance/LConn2 -- Activation Switches/LConn5 -- Controlled Current Source1/RConn1
  Voltage Measurement/LConn2 -- Activation Switches/RConn3 -- Voltage Measurement1/LConn2 -- Current Measurement2/LConn1
  Controlled Voltage Source/LConn1 -- Activation Switches/LConn2 -- Controlled Voltage Source1/RConn1
  Voltage Measurement1/LConn1 -- Activation Switches/RConn2 -- Current Measurement1/LConn1
  Current Measurement/RConn1 -- A/RConn1
  Current Measurement1/RConn1 -- B/RConn1
  C/RConn1 -- Current Measurement2/RConn1
  Controlled Voltage Source/RConn1 -- Activation Switches/LConn1
  Activation Switches/LConn3 -- Controlled Voltage Source1/LConn1

== system motorcontroller/Motor/Torque limitation ==
  N rad/s : Inport
  Torque : Inport  Port=2
  Abs1 : Abs  SaturateOnIntegerOverflow=on
  Gain : Gain  Gain=-1
  Saturation Dynamic : simulink/Discontinuities/Saturation Dynamic  OutMin=[]  OutMax=[]  OutDataTypeStr=Inherit: Same as second input  OutDataType=sfix(16)  OutScaling=2^-10  DoSatur=off
  Torque vs speed profile : Lookup  InputValues=[0 1200 2000 3000 4000 5000 6000]*pi/30  Table=[400 400 225 150 100 80 70]  LookUpMeth=Interpolation-Use End Values
  torque : Outport
  wires:
  N rad/s/1 -> Abs1/1
  Abs1/1 -> Torque vs speed profile/1
  Torque vs speed profile/1 -> Saturation Dynamic/1, Gain/1
  Saturation Dynamic/1 -> torque/1
  Torque/1 -> Saturation Dynamic/2
  Gain/1 -> Saturation Dynamic/3

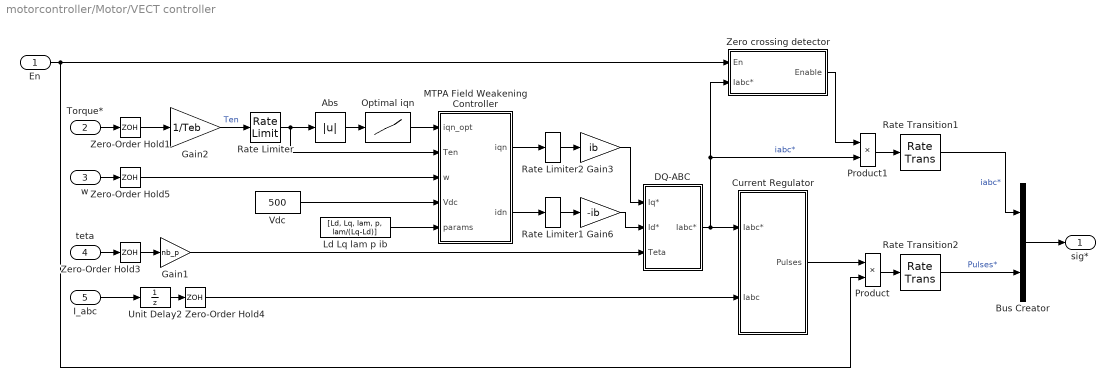
== system motorcontroller/Motor/VECT controller ==
  En : Inport
  Torque* : Inport  Port=2
  w : Inport  Port=3
  teta : Inport  Port=4
  I_abc : Inport  Port=5
  Abs : Abs
  Bus Creator : BusCreator  Inputs=2
  Current Regulator : Subsystem
  DQ-ABC : Subsystem
  Gain1 : Gain  Gain=nb_p  SaturateOnIntegerOverflow=on  OutDataTypeStr=Inherit: Same as input  ParamDataTypeStr=Inherit: Same as input
  Gain2 : Gain  Gain=1/Teb  SaturateOnIntegerOverflow=on  OutDataTypeStr=Inherit: Same as input  ParamDataTypeStr=Inherit: Same as input
  Gain3 : Gain  Gain=ib  SaturateOnIntegerOverflow=on  OutDataTypeStr=Inherit: Same as input  ParamDataTypeStr=Inherit: Same as input
  Gain6 : Gain  Gain=-ib  SaturateOnIntegerOverflow=on  OutDataTypeStr=Inherit: Same as input  ParamDataTypeStr=Inherit: Same as input
  Ld Lq lam p ib : Constant  Value=[Ld, Lq, lam, p, lam/(Lq-Ld)]
  MTPA Field Weakening Controller : MATLAB Function  TreatAsAtomicUnit=on  SystemSampleTime=Ts_vect
  Optimal iqn : Lookup  InputValues=ten  Table=iqn
  Product : Product  RndMeth=Zero
  Product1 : Product  RndMeth=Zero
  Rate Limiter : RateLimiter  RisingSlewLimit=10  FallingSlewLimit=-10  LinearizeAsGain=off
  Rate Limiter1 : RateLimiter  RisingSlewLimit=100  FallingSlewLimit=-100  SampleTimeMode=inherited
  Rate Limiter2 : RateLimiter  RisingSlewLimit=100  FallingSlewLimit=-100  SampleTimeMode=inherited
  Rate Transition1 : RateTransition
  Rate Transition2 : RateTransition
  Unit Delay2 : UnitDelay  SampleTime=-1
  Vdc : Constant  Value=500
  Zero crossing detector : Subsystem
  Zero-Order Hold{1,3..5} (4 alike) : ZeroOrderHold  SampleTime=Ts_vect
  sig* : Outport
  wires:
  Unit Delay2/1 -> Zero-Order Hold4/1
  Zero-Order Hold4/1 -> Current Regulator/2(Iabc)
  teta/1 -> Zero-Order Hold3/1
  Zero-Order Hold3/1 -> Gain1/1
  Gain1/1 -> DQ-ABC/3(Teta)
  DQ-ABC/1(Iabc*) -> Current Regulator/1(Iabc*), Zero crossing detector/2(Iabc*), Product1/2  "iabc*"
  I_abc/1 -> Unit Delay2/1
  Torque*/1 -> Zero-Order Hold1/1
  Gain3/1 -> DQ-ABC/1("Iq* ")
  Gain6/1 -> DQ-ABC/2("Id* ")
  Zero-Order Hold1/1 -> Gain2/1
  w/1 -> Zero-Order Hold5/1
  MTPA Field Weakening Controller/2(idn) -> Rate Limiter1/1
  Gain2/1 -> Rate Limiter/1  "Ten"
  Zero-Order Hold5/1 -> MTPA Field Weakening Controller/3(w)
  Ld Lq lam p ib/1 -> MTPA Field Weakening Controller/5(params)
  MTPA Field Weakening Controller/1(iqn) -> Rate Limiter2/1
  Optimal iqn/1 -> MTPA Field Weakening Controller/1(iqn_opt)
  Abs/1 -> Optimal iqn/1
  Vdc/1 -> MTPA Field Weakening Controller/4(Vdc)
  Bus Creator/1 -> sig*/1
  Rate Transition2/1 -> Bus Creator/2  "Pulses*"
  Rate Transition1/1 -> Bus Creator/1  "iabc*"
  Current Regulator/1(Pulses) -> Product/1
  Product/1 -> Rate Transition2/1
  Product1/1 -> Rate Transition1/1
  Zero crossing detector/1(Enable) -> Product1/1
  En/1 -> Zero crossing detector/1(En), Product/2
  Rate Limiter2/1 -> Gain3/1
  Rate Limiter1/1 -> Gain6/1
  Rate Limiter/1 -> Abs/1, MTPA Field Weakening Controller/2(Ten)

== system motorcontroller/DC//DC Converter/Bus DC controller/Current controller DISCRETE1 ==
  UBus : Inport
  Uref : Inport  Port=2
  Clock1 : Clock
  Compare To Constant1 : simulink/Logic and Bit Operations/Compare To Constant  relop=>  const=0.01  OutDataTypeStr=uint8  ZeroCross=off
  Ctrl sat. : Saturate  UpperLimit=0.95  LowerLimit=-0.95
  Discrete-Time Integrator : DiscreteIntegrator  IntegratorMethod=Integration: Trapezoidal  SampleTime=Ts  LimitOutput=on  UpperSaturationLimit=1  LowerSaturationLimit=-1
  Integral gain : Gain  Gain=Ki  SaturateOnIntegerOverflow=on  OutDataTypeStr=Inherit: Same as input  ParamDataTypeStr=Inherit: Same as input
  Product1 : Product  RndMeth=Zero
  Proportional gain : Gain  Gain=Kp  SaturateOnIntegerOverflow=on  OutDataTypeStr=Inherit: Same as input  ParamDataTypeStr=Inherit: Same as input
  Sum1 : Sum  Inputs=+-  SaturateOnIntegerOverflow=on  InputSameDT=on  OutDataTypeStr=Inherit: Same as first input
  Sum2 : Sum  SaturateOnIntegerOverflow=on  InputSameDT=on  OutDataTypeStr=Inherit: Same as first input
  Ec : Outport  InitialOutput=0
  wires:
  Sum2/1 -> Ctrl sat./1
  Discrete-Time Integrator/1 -> Sum2/2
  Uref/1 -> Sum1/2
  UBus/1 -> Sum1/1
  Integral gain/1 -> Discrete-Time Integrator/1
  Proportional gain/1 -> Sum2/1
  Ctrl sat./1 -> Ec/1
  Sum1/1 -> Product1/1
  Clock1/1 -> Compare To Constant1/1
  Compare To Constant1/1 -> Product1/2
  Product1/1 -> Integral gain/1, Proportional gain/1

== system motorcontroller/DC//DC Converter/Bus DC controller/Duty Cycles ==
  Ec : Inport
  Add : Sum  Inputs=+-
  Bus Creator2 : BusCreator  Inputs=2
  Constant : Constant
  Duty Cycle : Fcn  Expr=0.5*(u[1]+1)
  dc : Outport
  wires:
  Bus Creator2/1 -> dc/1
  Ec/1 -> Duty Cycle/1
  Constant/1 -> Add/1
  Add/1 -> Bus Creator2/2  "IGBT 2"
  Duty Cycle/1 -> Bus Creator2/1, Add/2  "IGBT I"

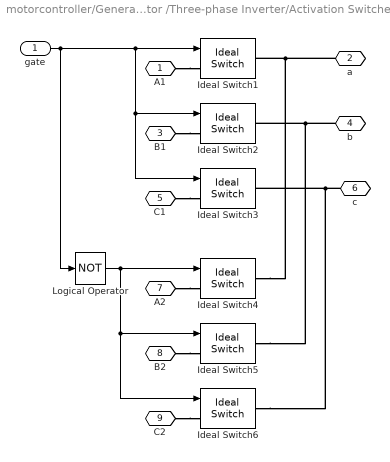
== system motorcontroller/Generator /Three-phase Inverter/Activation Switches ==
  gate : Inport
  Ideal Switch1 : powerlib/Power Electronics/Ideal Switch  Ron=2*Ron  Lon=0  IC=1  Rs=1e6  Cs=inf  Measurements=off
  Ideal Switch2 : powerlib/Power Electronics/Ideal Switch  Ron=2*Ron  Lon=0  IC=1  Rs=1e6  Cs=inf  Measurements=off
  Ideal Switch3 : powerlib/Power Electronics/Ideal Switch  Ron=2*Ron  Lon=0  IC=1  Rs=1e6  Cs=inf  Measurements=off
  Ideal Switch4 : powerlib/Power Electronics/Ideal Switch  Ron=2*Ron  Lon=0  IC=0  Rs=1e6  Cs=inf  Measurements=off
  Ideal Switch5 : powerlib/Power Electronics/Ideal Switch  Ron=2*Ron  Lon=0  IC=0  Rs=1e6  Cs=inf  Measurements=off
  Ideal Switch6 : powerlib/Power Electronics/Ideal Switch  Ron=2*Ron  Lon=0  IC=0  Rs=1e6  Cs=inf  Measurements=off
  Logical Operator : Logic  Operator=NOT  AllPortsSameDT=off  OutDataTypeStr=boolean
  A1 : PMIOPort  Port=1  Side=Left
  a : PMIOPort  Port=2  Side=Right
  B1 : PMIOPort  Port=3  Side=Left
  b : PMIOPort  Port=4  Side=Right
  C1 : PMIOPort  Port=5  Side=Left
  c : PMIOPort  Port=6  Side=Right
  A2 : PMIOPort  Port=7  Side=Left
  B2 : PMIOPort  Port=8  Side=Left
  C2 : PMIOPort  Port=9  Side=Left
  wires:
  Logical Operator/1 -> Ideal Switch6/1, Ideal Switch5/1, Ideal Switch4/1
  gate/1 -> Logical Operator/1, Ideal Switch3/1, Ideal Switch2/1, Ideal Switch1/1
  connections:
  C2/RConn1 -- Ideal Switch6/LConn1
  B2/RConn1 -- Ideal Switch5/LConn1
  A2/RConn1 -- Ideal Switch4/LConn1
  c/RConn1 -- Ideal Switch6/RConn1 -- Ideal Switch3/RConn1
  C1/RConn1 -- Ideal Switch3/LConn1
  b/RConn1 -- Ideal Switch5/RConn1 -- Ideal Switch2/RConn1
  B1/RConn1 -- Ideal Switch2/LConn1
  Ideal Switch4/RConn1 -- a/RConn1 -- Ideal Switch1/RConn1
  A1/RConn1 -- Ideal Switch1/LConn1

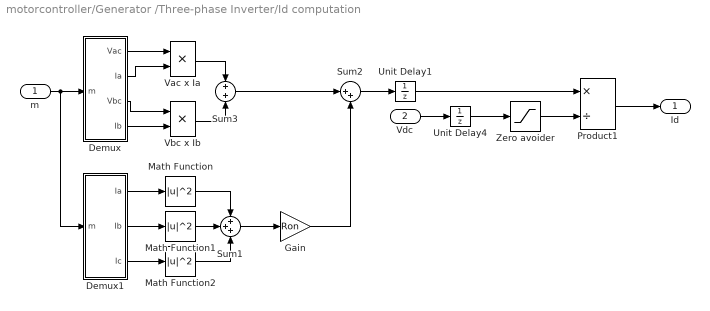
== system motorcontroller/Generator /Three-phase Inverter/Id computation ==
  m : Inport
  Vdc : Inport  Port=2
  Demux : Subsystem
  Demux1 : Subsystem
  Gain : Gain  Gain=Ron
  Math Function : Math  Operator=magnitude^2  SaturateOnIntegerOverflow=on
  Math Function1 : Math  Operator=magnitude^2  SaturateOnIntegerOverflow=on
  Math Function2 : Math  Operator=magnitude^2  SaturateOnIntegerOverflow=on
  Product1 : Product  Inputs=*/  SaturateOnIntegerOverflow=on  OutDataTypeStr=Inherit: Same as first input
  Sum1 : Sum  Inputs=+++  SaturateOnIntegerOverflow=on
  Sum2 : Sum  Inputs=|++  SaturateOnIntegerOverflow=on
  Sum3 : Sum  SaturateOnIntegerOverflow=on
  Unit Delay1 : UnitDelay  SampleTime=Ts
  Unit Delay4 : UnitDelay  InitialCondition=1  SampleTime=Ts
  Vac x Ia : Product  SaturateOnIntegerOverflow=on  OutDataTypeStr=Inherit: Same as first input
  Vbc x Ib : Product  SaturateOnIntegerOverflow=on  OutDataTypeStr=Inherit: Same as first input
  Zero avoider : Saturate  UpperLimit=inf  LowerLimit=1
  Id : Outport
  wires:
  Zero avoider/1 -> Product1/2
  Product1/1 -> Id/1
  Gain/1 -> Sum2/2
  Demux/3(Vbc) -> Vbc x Ib/1
  Demux/4(Ib) -> Vbc x Ib/2
  Demux/2(Ia) -> Vac x Ia/2
  Demux/1(Vac) -> Vac x Ia/1
  Vdc/1 -> Unit Delay4/1
  Vbc x Ib/1 -> Sum3/2
  Vac x Ia/1 -> Sum3/1
  m/1 -> Demux/1(m), Demux1/1(m)
  Unit Delay1/1 -> Product1/1
  Unit Delay4/1 -> Zero avoider/1
  Demux1/1(Ia) -> Math Function/1
  Demux1/2(Ib) -> Math Function1/1
  Demux1/3(Ic) -> Math Function2/1
  Math Function1/1 -> Sum1/2
  Math Function/1 -> Sum1/1
  Math Function2/1 -> Sum1/3
  Sum1/1 -> Gain/1
  Sum3/1 -> Sum2/1
  Sum2/1 -> Unit Delay1/1

== system motorcontroller/Generator /Three-phase Inverter/Limit detection ==
  note: Low pass filter
  note: Low pass filter
  note: Limit = 1 saturation mode (voltage mode)
      | Limit = 0 normal mode (current mode)
  Vcc : Inport
  ctrl : Inport  Port=2
  Bus Selector1 : BusSelector  OutputSignals=m.Stator current is_d (A),m.Stator current is_q (A),m.Rotor speed wm (rad/s)  OutputAsBus=on
  Discrete Transfer Fcn1 : DiscreteTransferFcn  Numerator=[1-exp(-Ts*Fcs*2*pi)]  Denominator=[1 -exp(-Ts*Fcs*2*pi)]  SampleTime=Ts
  Discrete Transfer Fcn3 : DiscreteTransferFcn  Numerator=[1-exp(-Ts*Fcs*2*pi)]  Denominator=[1 -exp(-Ts*Fcs*2*pi)]  SampleTime=Ts
  Gain1 : Gain  Gain=0.9  SaturateOnIntegerOverflow=on  OutDataTypeStr=Inherit: Same as input  ParamDataTypeStr=Inherit: Same as input
  "Internal Vcc " : Fcn  Expr=pi/2*sqrt((Resistance*u(1)-Lq*p*u(3)*u(2))^2+(Resistance*u(2)+Ld*p*u(3)*u(1)+Flux*p*u(3))^2)
  Relational Operator : RelationalOperator  Operator=>  OutDataTypeStr=boolean
  Relational Operator2 : RelationalOperator  Operator=<  OutDataTypeStr=boolean
  S-R Flip-Flop : simulink_extras/Flip Flops/S-R Flip-Flop  initial_condition=0
  Terminator : Terminator
  Limit : Outport
  wires:
  S-R Flip-Flop/2 -> Terminator/1
  Discrete Transfer Fcn3/1 -> Relational Operator/2, Gain1/1
  Gain1/1 -> Relational Operator2/2
  Discrete Transfer Fcn1/1 -> Relational Operator2/1, Relational Operator/1
  "Internal Vcc "/1 -> Discrete Transfer Fcn1/1
  Bus Selector1/1 -> "Internal Vcc "/1
  ctrl/1 -> Bus Selector1/1
  S-R Flip-Flop/1 -> Limit/1
  Relational Operator2/1 -> S-R Flip-Flop/2
  Relational Operator/1 -> S-R Flip-Flop/1
  Vcc/1 -> Discrete Transfer Fcn3/1

== system motorcontroller/Generator /Three-phase Inverter/Output Resistance correction ==
  note: Vabc
  ctrl : Inport
  1/R : Gain  Gain=1/(100*Resistance)  SaturateOnIntegerOverflow=on  OutDataTypeStr=Inherit: Same as input  ParamDataTypeStr=Inherit: Same as input
  Bus Selector1 : BusSelector  OutputSignals=m.Stator voltage Vs_d (V),m.Stator voltage Vs_q (V),m.Rotor angle thetam (rad)
  Constant : Constant  Value=0
  Discrete Transfer Fcn1 : DiscreteTransferFcn  Numerator=[1-exp(-Ts/.001)]  Denominator=[1 -exp(-Ts/.001)]  SampleTime=Ts
  Discrete Transfer Fcn2 : DiscreteTransferFcn  Numerator=[1-exp(-Ts/.001)]  Denominator=[1 -exp(-Ts/.001)]  SampleTime=Ts
  Fcn : Fcn  Expr=sin(u)
  Fcn1 : Fcn  Expr=cos(u)
  Mux4 : Mux  Inputs=3
  Mux5 : Mux  Inputs=2
  dq0_to_abc Transformation : powerlib_extras/Measurements/dq0_to_abc Transformation
  poles : Gain  Gain=p  SaturateOnIntegerOverflow=on  OutDataTypeStr=Inherit: Same as input  ParamDataTypeStr=Inherit: Same as input
  "Iabc_r " : Outport
  wires:
  poles/1 -> Fcn/1, Fcn1/1
  Bus Selector1/3 -> poles/1  "<Rotor angle thetam (rad)>"
  Discrete Transfer Fcn1/1 -> Mux4/1
  Discrete Transfer Fcn2/1 -> Mux4/2
  dq0_to_abc Transformation/1 -> 1/R/1
  Constant/1 -> Mux4/3
  Mux5/1 -> dq0_to_abc Transformation/2
  Fcn1/1 -> Mux5/2
  Fcn/1 -> Mux5/1
  Mux4/1 -> dq0_to_abc Transformation/1
  ctrl/1 -> Bus Selector1/1
  Bus Selector1/1 -> Discrete Transfer Fcn1/1  "<Stator voltage Vs_d (V)>"
  Bus Selector1/2 -> Discrete Transfer Fcn2/1  "<Stator voltage Vs_q (V)>"
  1/R/1 -> "Iabc_r "/1

== system motorcontroller/Generator /VECT/Current Regulator ==
  Iabc* : Inport
  Iabc : Inport  Port=2
  Demux1 : Demux  Outputs=3
  Demux2 : Demux  Outputs=3
  Mux1 : Mux  Inputs=2
  Relay : Relay  OnSwitchValue=0  OffSwitchValue=0
  Relay1 : Relay  OnSwitchValue=0  OffSwitchValue=0
  Relay2 : Relay  OnSwitchValue=0  OffSwitchValue=0
  Sum : Sum  Inputs=-+  SaturateOnIntegerOverflow=on  InputSameDT=on  OutDataTypeStr=Inherit: Same as first input
  Sum1 : Sum  Inputs=-+  SaturateOnIntegerOverflow=on  InputSameDT=on  OutDataTypeStr=Inherit: Same as first input
  Sum2 : Sum  Inputs=-+  SaturateOnIntegerOverflow=on  InputSameDT=on  OutDataTypeStr=Inherit: Same as first input
  Sum3 : Sum  Inputs=+-
  Sum4 : Sum  Inputs=+-
  Pulses : Outport  InitialOutput=0
  wires:
  Sum4/1 -> Mux1/2
  Sum3/1 -> Mux1/1
  Relay2/1 -> Sum4/2
  Relay1/1 -> Sum4/1, Sum3/2
  Relay/1 -> Sum3/1
  Iabc*/1 -> Demux2/1
  Demux2/1 -> Sum/2
  Demux2/2 -> Sum1/2
  Demux2/3 -> Sum2/2
  Demux1/3 -> Sum2/1
  Sum2/1 -> Relay2/1
  Iabc/1 -> Demux1/1
  Mux1/1 -> Pulses/1
  Demux1/2 -> Sum1/1
  Demux1/1 -> Sum/1
  Sum1/1 -> Relay1/1
  Sum/1 -> Relay/1
